simulink model "FOC_PIL_StateMch_top"  (R2020b)
settings: Solver=FixedStepAuto  StartTime=0.0  StopTime=4  FixedStep=Ts_simscape  RelTol=1e-3
values from neighbouring files (symbols this model uses):
  Tctr = 0.0000625    (= 6.25e-05)    [FOC_Config.m]
undefined symbols (not defined in the file or in its folder): motor, NBits
libraries: fl_lib x51, nesl_utility x15, ee_lib x14, msbAdcArchitectures x4, dspsigops x4, simulink x3
settings Model: Creator=k  LastModifiedBy=k

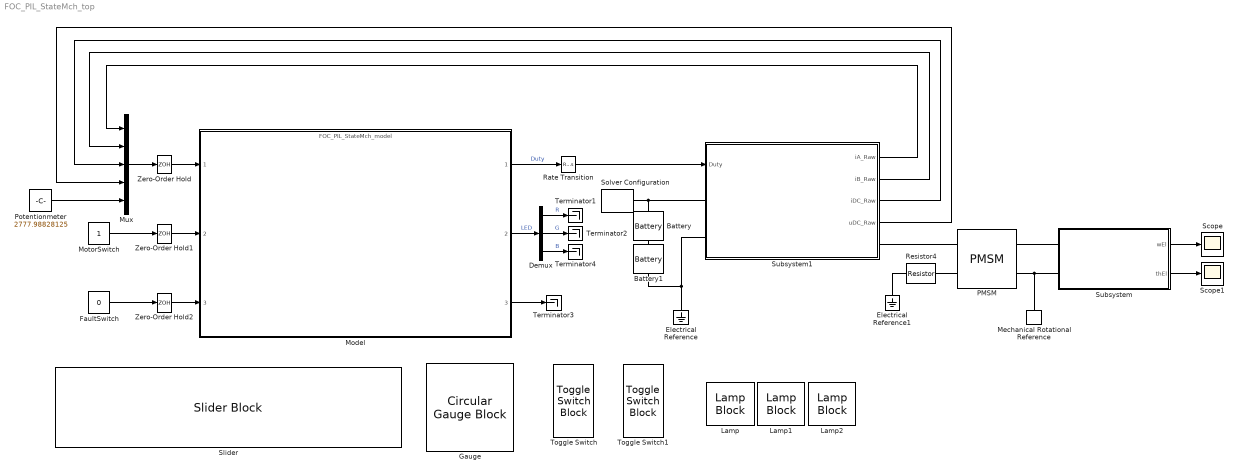
== system FOC_PIL_StateMch_top ==
  Battery : ee_lib/Sources/Battery  Vnom=motor.DC/2 V  prm_dir=1  R1_dis=2 Ohm  R1_ch=2 Ohm  R1=0.2 Ohm  prm_AH=1  AH=50 hr*A  V1=11.5 V  AH1=25 hr*A  prm_R2=1  R2=2000 Ohm  prm_dyn=1  Rp1=0.005 Ohm  tau1=30 s  Rp2=0.005 Ohm  tau2=30 s  Rp3=0.005 Ohm  tau3=30 s  Rp4=0.005 Ohm  tau4=30 s  Rp5=0.005 Ohm  tau5=30 s  prm_fade=1  N_fade=100  AH_fade=45 hr*A  R1_fade=2.02 Ohm  R1_ch_fade=2.02 Ohm  V1_fade=10.35 V  i_specify=off  i_priority=None  i=0 A  i_nominal_specify=off  i_nominal_unit=A  i_nominal_value=1  v_specify=off  v_priority=None  v=0 V  v_nominal_specify=off  v_nominal_unit=V  v_nominal_value=1  charge_specify=off  charge_priority=High  charge=50 hr*A  charge_nominal_specify=off  charge_nominal_unit=hr*A  charge_nominal_value=1  num_cycles_specify=off  num_cycles_priority=High  num_cycles=0  num_cycles_nominal_specify=off  num_cycles_nominal_unit=1  num_cycles_nominal_value=1  thermal_mass=30000 J/K  Tmeas=298.15 K  Vnom_T2=12 V  R1_T2=2.2 Ohm  R1_T2_dis=2.2 Ohm  R1_T2_ch=2.2 Ohm  V1_T2=11.4 V  R2_T2=2200 Ohm  Rp1_T2=0.005 Ohm  tau1_T2=30 s  Rp2_T2=0.005 Ohm  tau2_T2=30 s  Rp3_T2=0.005 Ohm  tau3_T2=30 s  Rp4_T2=0.005 Ohm  tau4_T2=30 s  Rp5_T2=0.005 Ohm  tau5_T2=30 s  Tmeas2=273.15 K  temperature_specify=off  temperature_priority=High  temperature=298.15 K  temperature_nominal_specify=off  temperature_nominal_unit=K  temperature_nominal_value=1
  Battery1 : ee_lib/Sources/Battery  Vnom=motor.DC/2 V  prm_dir=1  R1_dis=2 Ohm  R1_ch=2 Ohm  R1=0.2 Ohm  prm_AH=1  AH=50 hr*A  V1=11.5 V  AH1=25 hr*A  prm_R2=1  R2=2000 Ohm  prm_dyn=1  Rp1=0.005 Ohm  tau1=30 s  Rp2=0.005 Ohm  tau2=30 s  Rp3=0.005 Ohm  tau3=30 s  Rp4=0.005 Ohm  tau4=30 s  Rp5=0.005 Ohm  tau5=30 s  prm_fade=1  N_fade=100  AH_fade=45 hr*A  R1_fade=2.02 Ohm  R1_ch_fade=2.02 Ohm  V1_fade=10.35 V  i_specify=off  i_priority=None  i=0 A  i_nominal_specify=off  i_nominal_unit=A  i_nominal_value=1  v_specify=off  v_priority=None  v=0 V  v_nominal_specify=off  v_nominal_unit=V  v_nominal_value=1  charge_specify=off  charge_priority=High  charge=50 hr*A  charge_nominal_specify=off  charge_nominal_unit=hr*A  charge_nominal_value=1  num_cycles_specify=off  num_cycles_priority=High  num_cycles=0  num_cycles_nominal_specify=off  num_cycles_nominal_unit=1  num_cycles_nominal_value=1  thermal_mass=30000 J/K  Tmeas=298.15 K  Vnom_T2=12 V  R1_T2=2.2 Ohm  R1_T2_dis=2.2 Ohm  R1_T2_ch=2.2 Ohm  V1_T2=11.4 V  R2_T2=2200 Ohm  Rp1_T2=0.005 Ohm  tau1_T2=30 s  Rp2_T2=0.005 Ohm  tau2_T2=30 s  Rp3_T2=0.005 Ohm  tau3_T2=30 s  Rp4_T2=0.005 Ohm  tau4_T2=30 s  Rp5_T2=0.005 Ohm  tau5_T2=30 s  Tmeas2=273.15 K  temperature_specify=off  temperature_priority=High  temperature=298.15 K  temperature_nominal_specify=off  temperature_nominal_unit=K  temperature_nominal_value=1
  Demux : Demux  Outputs=3
  Electrical Reference : fl_lib/Electrical/Electrical Elements/Electrical Reference
  Electrical Reference1 : fl_lib/Electrical/Electrical Elements/Electrical Reference
  FaultSwitch : Constant  Value=0  OutDataTypeStr=boolean
  Gauge : CircularGaugeBlock  ScaleMin=-3.14  ScaleMax=3.14  TickInterval=1.57
  Lamp : LampBlock
  Lamp1 : LampBlock
  Lamp2 : LampBlock
  Mechanical Rotational Reference : fl_lib/Mechanical/Rotational Elements/Mechanical Rotational Reference
  Model : ModelReference  ModelNameDialog=FOC_PIL_StateMch_model.slx  SimulationMode=Processor-in-the-loop (PIL)  ModelReferenceVersion=1.590
  MotorSwitch : Constant  OutDataTypeStr=boolean
  Mux : Mux  Inputs=5
  PMSM : ee_lib/Electromechanical/Permanent Magnet/PMSM  winding_type=ee.enum.statorconnection.wye  machine_param=ee.enum.pmsm.parameterization.constant  nPolePairs=motor.Prs  pmflux_param=ee.enum.pmflux.fluxlinkage  pm_flux_linkage=motor.Flux Wb  torque_constant=0.18 N*m/A  back_emf_constant=0.18 V/(rad/s)  stator_param=ee.enum.statorparam.LdLqL0  Ld=motor.Ld H  Lq=motor.Lq H  idVec=[-200, 0, 200] A  iqVec=[-200, 0, 200] A  LdMatrix=0.0002 * ones(3, 3) H  LqMatrix=0.0002 * ones(3, 3) H  PmMatrix=0.1 * ones(3, 3) Wb  ktMatrix=0.18 * ones(3, 3) N*m/A  keMatrix=0.18 * ones(3, 3) V/(rad/s)  L0=motor.L0 H  Ls=0.0002 H  Lm=-0.00002 H  Ms=0.00002 H  Rs=motor.Rs Ohm  zero_sequence=ee.enum.park.zerosequence.exclude  J=motor.J kg*m^2  lam=motor.B N*m/(rad/s)  axes_param=ee.enum.rotorangle.daxis  i_d_specify=off  i_d_priority=None  i_d=0 A  i_d_nominal_specify=off  i_d_nominal_unit=A  i_d_nominal_value=1  i_q_specify=off  i_q_priority=None  i_q=0 A  i_q_nominal_specify=off  i_q_nominal_unit=A  i_q_nominal_value=1  torque_specify=off  torque_priority=None  torque=0 N*m  torque_nominal_specify=off  torque_nominal_unit=N*m  torque_nominal_value=1  angular_velocity_specify=off  angular_velocity_priority=High  angular_velocity=0 rpm  angular_velocity_nominal_specify=off  angular_velocity_nominal_unit=rpm  angular_velocity_nominal_value=1  angular_position_specify=off  angular_position_priority=High  angular_position=0 deg  angular_position_nominal_specify=off  angular_position_nominal_unit=deg  angular_position_nominal_value=1  loss_param=ee.enum.ironloss.none  losses_oc=[0, 0, 0] W  losses_sc=[0, 0, 0] W  f_losses=60 Hz  Isc_losses=95 A  Tmeas=298.15 K  alpha=3.93e-3 1/K  alpha_flux=-0.001 1/K  stator_thermal_mass=100 J/K  rotor_thermal_mass=200 J/K  Rm_percent_rotor=90  Rd_percent_rotor=30  temperatureA_specify=off  temperatureA_priority=High  temperatureA=25 degC  temperatureA_nominal_specify=off  temperatureA_nominal_unit=degC  temperatureA_nominal_value=1  temperatureB_specify=off  temperatureB_priority=High  temperatureB=25 degC  temperatureB_nominal_specify=off  temperatureB_nominal_unit=degC  temperatureB_nominal_value=1  temperatureC_specify=off  temperatureC_priority=High  temperatureC=25 degC  temperatureC_nominal_specify=off  temperatureC_nominal_unit=degC  temperatureC_nominal_value=1  temperatureR_specify=off  temperatureR_priority=High  temperatureR=25 degC  temperatureR_nominal_specify=off  temperatureR_nominal_unit=degC  temperatureR_nominal_value=1
      settings: InternalSimscapePortConfiguration="{\"Bottom\":[],\"Left\":[{\"id\":\"N\",\"label\":\"~\",\"type\":\"foundation.electrical.three_phase\"},{\"id\":\"n\",\"label\":\"n\",\"type\":\"foundation.electrical.electrical\"}],\"Right\":[{\"id\":\"R\",\"label\":\"R\",\"type\":\"foundation.mechanical.rotational.rotational\"},{\"id\":\"C\",\"label\":\"C\",\"type\":\"foundation.mechanical.rotational.rotational\"}],\"Top\":[]}"
  Potentionmeter : Constant  Value=2777.98828125  OutDataTypeStr=uint16
  Rate Transition : RateTransition
  Resistor4 : fl_lib/Electrical/Electrical Elements/Resistor  R=1e6 Ohm  i_specify=off  i_priority=None  i=0 A  i_nominal_specify=off  i_nominal_unit=A  i_nominal_value=1  v_specify=off  v_priority=None  v=0 V  v_nominal_specify=off  v_nominal_unit=V  v_nominal_value=1
  Scope : Scope
  Scope1 : Scope
  Slider : SliderBlock  ScaleMax=4095
  Solver Configuration : nesl_utility/Solver Configuration  PhysicalDomain=network_engine_domain  SubClassName=solver  LeftPortType=input  RightPortType=generic  Tones=[]  Harmonics=[]  SimulateNoise=off  Profile=off  UseLocalSampling=off  EnableSwitchedLinearOptims=on  FrequencyDomain=off  UseCCode=off  RelTol=0.001  AbsTol=1e-06  MinStep=1e-09  ToWorkspace=off  RevertToSquareIcSolve=off  NumHomotopyIterations=100  PhasorMode=off  PhasorModeNumHarmonics=1  DoDC=off  ResidualTolerance=1e-09  UseLocalSolver=off  LocalSolverChoice=NE_BACKWARD_EULER_ADVANCER  LocalSolverSampleTime=0.001  DoFixedCost=off  MaxNonlinIter=3  MaxModeIter=2  ComputeImpulses=off  ImpulseIterations=2  LinearAlgebra=auto  EquationFormulation=NE_TIME_EF  DelaysMemoryBudget=1024  AutomaticFiltering=on  FilteringTimeConstant=0.001  PartitionStorageMethod=AS_NEEDED  PartitionMemoryBudget=1024  PartitionMethod=ROBUST
  Subsystem : Subsystem
  Subsystem1 : Subsystem
  Terminator{1..4} (4 alike) : Terminator
  Toggle Switch : ToggleSwitchBlock
      settings: Values={{'Off', 'On'}, [0 1]}
  Toggle Switch1 : ToggleSwitchBlock
      settings: Values={{'Off', 'On'}, [0 1]}
  Zero-Order Hold : ZeroOrderHold  SampleTime=Tctr
  Zero-Order Hold1 : ZeroOrderHold  SampleTime=Tctr
  Zero-Order Hold2 : ZeroOrderHold  SampleTime=Tctr
  wires:
  Model/2 -> Demux/1  "LED"
  Model/3 -> Terminator3/1
  Model/1 -> Rate Transition/1  "Duty"
  Subsystem1/3(" iDC_Raw") -> Mux/3
  Mux/1 -> Zero-Order Hold/1
  Subsystem1/1(" iA_Raw") -> Mux/1
  Subsystem1/2(" iB_Raw") -> Mux/2
  Subsystem1/4(" uDC_Raw") -> Mux/4
  Potentionmeter/1 -> Mux/5
  MotorSwitch/1 -> Zero-Order Hold1/1
  FaultSwitch/1 -> Zero-Order Hold2/1
  Zero-Order Hold/1 -> Model/1
  Zero-Order Hold1/1 -> Model/2
  Zero-Order Hold2/1 -> Model/3
  Rate Transition/1 -> Subsystem1/1(Duty)
  Subsystem/1(wEl) -> Scope/1
  Subsystem/2(thEl) -> Scope1/1
  Demux/1 -> Terminator1/1  "R"
  Demux/2 -> Terminator2/1  "G"
  Demux/3 -> Terminator4/1  "B"
  connections:
  Subsystem1/LConn2 -- Electrical Reference/LConn1 -- Battery1/RConn1
  Subsystem1/LConn1 -- Solver Configuration/RConn1 -- Battery/LConn1
  Resistor4/RConn1 -- Electrical Reference1/LConn1
  Resistor4/LConn1 -- PMSM/LConn2
  Battery1/LConn1 -- Battery/RConn1
  PMSM/RConn2 -- Mechanical Rotational Reference/LConn1 -- Subsystem/LConn2
  Subsystem1/RConn1 -- PMSM/LConn1
  Subsystem/LConn1 -- PMSM/RConn1

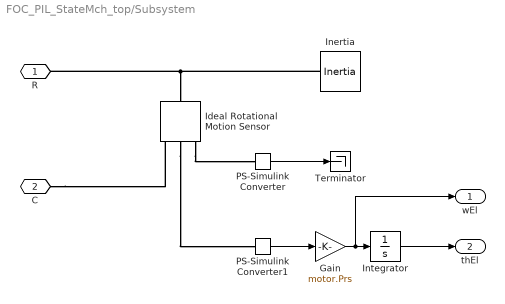
== system FOC_PIL_StateMch_top/Subsystem ==
  Gain : Gain  Gain=motor.Prs
  Ideal Rotational Motion Sensor : fl_lib/Mechanical/Mechanical Sensors/Ideal Rotational Motion Sensor  wrap_angle=simscape.enum.onoff.on  offset=0 rad
  Inertia : fl_lib/Mechanical/Rotational Elements/Inertia  inertia=0.000001 kg*m^2  num_ports=foundation.enum.numPorts2.one  w_specify=off  w_priority=High  w=0 rad/s  w_nominal_specify=off  w_nominal_unit=rad/s  w_nominal_value=1  t_specify=off  t_priority=None  t=0 N*m  t_nominal_specify=off  t_nominal_unit=N*m  t_nominal_value=1
  Integrator : Integrator  WrapState=on
  PS-Simulink Converter : nesl_utility/PS-Simulink Converter  PhysicalDomain=network_engine_domain  SubClassName=ps_output  LeftPortType=input  RightPortType=output  PseudoPeriodic=off  Frequencies=[]  Unit=inherit  AffineConversion=off
  PS-Simulink Converter1 : nesl_utility/PS-Simulink Converter  PhysicalDomain=network_engine_domain  SubClassName=ps_output  LeftPortType=input  RightPortType=output  PseudoPeriodic=off  Frequencies=[]  Unit=inherit  AffineConversion=off
  Terminator : Terminator
  R : PMIOPort  Side=Left
  C : PMIOPort  Port=2  Side=Left
  wEl : Outport
  thEl : Outport  Port=2
  wires:
  PS-Simulink Converter1/1 -> Gain/1
  Integrator/1 -> thEl/1
  PS-Simulink Converter/1 -> Terminator/1
  Gain/1 -> wEl/1, Integrator/1
  connections:
  C/RConn1 -- Ideal Rotational Motion Sensor/RConn1
  Inertia/LConn1 -- R/RConn1 -- Ideal Rotational Motion Sensor/LConn1
  Ideal Rotational Motion Sensor/RConn2 -- PS-Simulink Converter1/LConn1
  Ideal Rotational Motion Sensor/RConn3 -- PS-Simulink Converter/LConn1

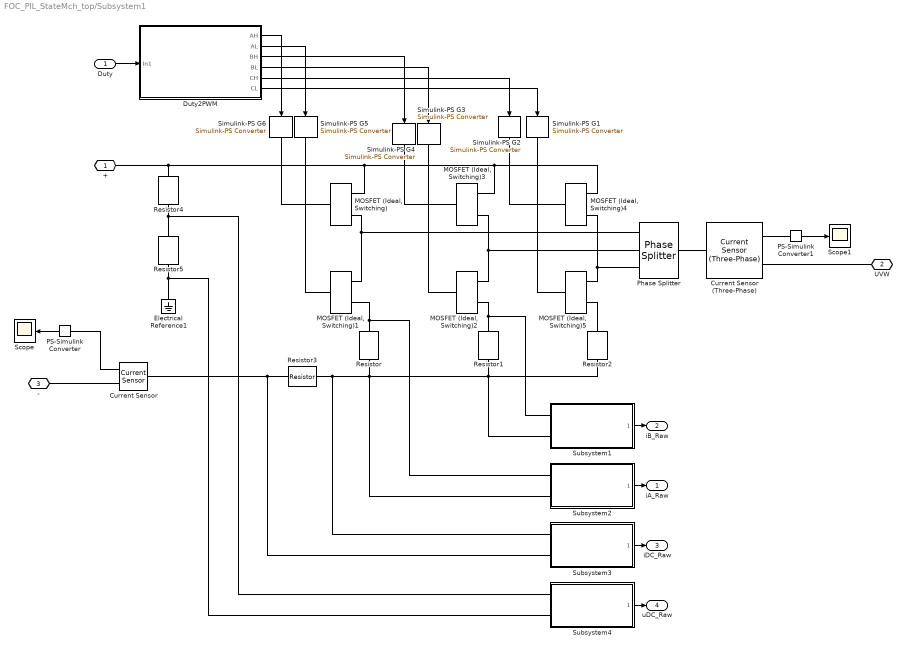
== system FOC_PIL_StateMch_top/Subsystem1 ==
  Duty : Inport
  Current Sensor : fl_lib/Electrical/Electrical Sensors/Current Sensor
  Current Sensor (Three-Phase) : ee_lib/Sensors & Transducers/Current Sensor (Three-Phase)
  Duty2PWM : Subsystem
  Electrical Reference1 : fl_lib/Electrical/Electrical Elements/Electrical Reference
  MOSFET (Ideal, Switching){,1..5} (6 alike) : ee_lib/Semiconductors & Converters/MOSFET (Ideal, Switching)  Rds=0.035 Ohm  Goff=1e-6 1/Ohm  Vth=0.5 V  diode_param=1  diode_Vf=0.8 V  diode_Ron=0.001 Ohm  diode_Goff=1e-5 1/Ohm  diode_C=50e-9 F  diode_iRM=-235 A  diode_iF=300 A  diode_idot=-50 A/us  diode_trr_param=1  diode_trr_factor=3  diode_trr=15 us  diode_Qrr=1500 s*uA  thermal_loss_option=ee.enum.converters.thermalLossOption.constantvalues  Von_data=[0, 1.1, 1.3, 1.45, 1.75, 2.25, 2.7; 0, 1, 1.15, 1.35, 1.7, 2.35, 3] V  Eon_data=[0, .29, 1.43, 2.86, 5.71, 13.14, 22.86; 0, .57, 2.63, 5.14, 10.29, 20.57, 30.29] * 1e-3 J  Eoff_data=[0, .21, 1.07, 2.14, 4.29, 9.86, 17.14; 0, .43, 1.97, 3.86, 7.71, 15.43, 22.71] * 1e-3 J  Tj=[298.15, 398.15] K  Iout_data=[0, 10, 50, 100, 200, 400, 600] A  Eon_scalar=22.86e-3 J  Eoff_scalar=17.14e-3 J  Voff=300 V  Iout_scalar=600 A  diodeModelType=ee.enum.converters.diodeModelType.pwl  diode_IfMat=[.07, .12, .19, 1.75, 4.24, 7.32, 11.2; .16, .3, .72, 2.14, 4.02, 6.35, 9.12] A  diode_TjVec=[25, 125] degC  diode_VfVec=[.5, .7, .9, 1.3, 1.7, 2.1, 2.5] V  thermal_network_parameterization=ee.enum.thermalNetworkTopology.external  Rth=[.03, .2] K/W  Rth_Foster=[.03, .2] K/W  thermal_mass_parameterization=ee.enum.thermalNetwork.timeconstant  thermal_mass=[3, 25] J/K  thermal_mass_Foster=[33, 50] J/K  thermal_time_constant=[.1, 5] s  thermal_time_constant_Foster=[1, 10] s  thermal_mass_initial_temperatures=[25, 25] degC  junction_thermal_mass=0.1 J/K  Tau=1e-4 s  vT_specify=off  vT_priority=None  vT=0 V  vT_nominal_specify=off  vT_nominal_unit=V  vT_nominal_value=1  Qj_specify=off  Qj_priority=None  Qj=0 W  Qj_nominal_specify=off  Qj_nominal_unit=W  Qj_nominal_value=1  junction_temperature_specify=off  junction_temperature_priority=None  junction_temperature=25 degC  junction_temperature_nominal_specify=off  junction_temperature_nominal_unit=degC  junction_temperature_nominal_value=1
  PS-Simulink Converter : nesl_utility/PS-Simulink Converter  PhysicalDomain=network_engine_domain  SubClassName=ps_output  LeftPortType=input  RightPortType=output  PseudoPeriodic=off  Frequencies=[]  Unit=inherit  AffineConversion=off
  PS-Simulink Converter1 : nesl_utility/PS-Simulink Converter  PhysicalDomain=network_engine_domain  SubClassName=ps_output  LeftPortType=input  RightPortType=output  PseudoPeriodic=off  Frequencies=[]  Unit=inherit  AffineConversion=off
  Phase Splitter : ee_lib/Connectors & References/Phase Splitter
      settings: SourceProductBaseCode=PS
  Resistor{,1..3} (4 alike) : fl_lib/Electrical/Electrical Elements/Resistor  R=0.01 Ohm  i_specify=off  i_priority=None  i=0 A  i_nominal_specify=off  i_nominal_unit=A  i_nominal_value=1  v_specify=off  v_priority=None  v=0 V  v_nominal_specify=off  v_nominal_unit=V  v_nominal_value=1
  Resistor4 : fl_lib/Electrical/Electrical Elements/Resistor  R=24000 Ohm  i_specify=off  i_priority=None  i=0 A  i_nominal_specify=off  i_nominal_unit=A  i_nominal_value=1  v_specify=off  v_priority=None  v=0 V  v_nominal_specify=off  v_nominal_unit=V  v_nominal_value=1
  Resistor5 : fl_lib/Electrical/Electrical Elements/Resistor  R=3000 Ohm  i_specify=off  i_priority=None  i=0 A  i_nominal_specify=off  i_nominal_unit=A  i_nominal_value=1  v_specify=off  v_priority=None  v=0 V  v_nominal_specify=off  v_nominal_unit=V  v_nominal_value=1
  Scope : Scope
  Scope1 : Scope
  Simulink-PS G{1..6} (6 alike) : nesl_utility/Simulink-PS Converter  PhysicalDomain=network_engine_domain  SubClassName=ps_input  LeftPortType=input  RightPortType=output  PseudoPeriodic=off  Frequencies=[]  NoiseDistribution=none  NoiseParameters=[]  Unit=1  AffineConversion=off  FilteringAndDerivatives=zero  SimscapeFilterOrder=1  InputFilterTimeConstant=1e-6  UdotUserProvided=0
      settings: SourceProductName=Utilities
  Subsystem1 : Subsystem
  Subsystem2 : Subsystem
  Subsystem3 : Subsystem
  Subsystem4 : Subsystem
  + : PMIOPort  Side=Left
  UVW : PMIOPort  Port=2  Side=Right
  - : PMIOPort  Port=3  Side=Left
  " iA_Raw" : Outport
  " iB_Raw" : Outport  Port=2
  " iDC_Raw" : Outport  Port=3
  " uDC_Raw" : Outport  Port=4
  wires:
  Subsystem3/1(" ") -> " iDC_Raw"/1
  Subsystem2/1(" ") -> " iA_Raw"/1
  Subsystem1/1(" ") -> " iB_Raw"/1
  Duty/1 -> Duty2PWM/1(In1)
  Duty2PWM/1(AH) -> Simulink-PS G6/1
  Duty2PWM/2(AL) -> Simulink-PS G5/1
  Duty2PWM/3(BH) -> Simulink-PS G4/1
  Duty2PWM/4(BL) -> Simulink-PS G3/1
  Duty2PWM/5(CH) -> Simulink-PS G2/1
  Duty2PWM/6(CL) -> Simulink-PS G1/1
  PS-Simulink Converter/1 -> Scope/1
  PS-Simulink Converter1/1 -> Scope1/1
  Subsystem4/1(" ") -> " uDC_Raw"/1
  connections:
  Subsystem3/LConn2 -- Resistor3/RConn1 -- Current Sensor/LConn1
  Simulink-PS G3/RConn1 -- "MOSFET (Ideal, Switching)2"/LConn1
  "MOSFET (Ideal, Switching)4"/RConn2 -- "MOSFET (Ideal, Switching)5"/RConn1 -- Phase Splitter/RConn3
  Phase Splitter/RConn1 -- "MOSFET (Ideal, Switching)"/RConn2 -- "MOSFET (Ideal, Switching)1"/RConn1
  Simulink-PS G4/RConn1 -- "MOSFET (Ideal, Switching)3"/LConn1
  Subsystem2/LConn2 -- Subsystem1/LConn2 -- Resistor1/RConn1 -- Resistor2/RConn1 -- Resistor/RConn1 -- Resistor3/LConn1 -- Subsystem3/LConn1
  "MOSFET (Ideal, Switching)2"/RConn2 -- Subsystem1/LConn1 -- Resistor1/LConn1
  +/RConn1 -- "MOSFET (Ideal, Switching)"/RConn1 -- "MOSFET (Ideal, Switching)3"/RConn1 -- "MOSFET (Ideal, Switching)4"/RConn1 -- Resistor4/LConn1
  Phase Splitter/RConn2 -- "MOSFET (Ideal, Switching)3"/RConn2 -- "MOSFET (Ideal, Switching)2"/RConn1
  Simulink-PS G6/RConn1 -- "MOSFET (Ideal, Switching)"/LConn1
  "MOSFET (Ideal, Switching)1"/RConn2 -- Resistor/LConn1 -- Subsystem2/LConn1
  Simulink-PS G2/RConn1 -- "MOSFET (Ideal, Switching)4"/LConn1
  Simulink-PS G5/RConn1 -- "MOSFET (Ideal, Switching)1"/LConn1
  "MOSFET (Ideal, Switching)5"/RConn2 -- Resistor2/LConn1
  Simulink-PS G1/RConn1 -- "MOSFET (Ideal, Switching)5"/LConn1
  Current Sensor (Three-Phase)/LConn1 -- Phase Splitter/LConn1
  Current Sensor/RConn2 -- -/RConn1
  Current Sensor/RConn1 -- PS-Simulink Converter/LConn1
  Current Sensor (Three-Phase)/RConn2 -- UVW/RConn1
  Current Sensor (Three-Phase)/RConn1 -- PS-Simulink Converter1/LConn1
  Resistor5/LConn1 -- Subsystem4/LConn1 -- Resistor4/RConn1
  Electrical Reference1/LConn1 -- Resistor5/RConn1 -- Subsystem4/LConn2

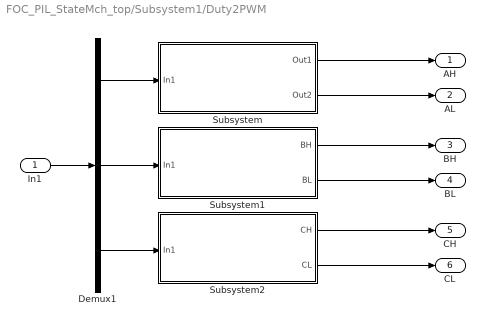
== system FOC_PIL_StateMch_top/Subsystem1/Duty2PWM ==
  In1 : Inport
  Demux1 : Demux  Outputs=3
  Subsystem : Subsystem
  Subsystem1 : Subsystem
  Subsystem2 : Subsystem
  AH : Outport
  AL : Outport  Port=2
  BH : Outport  Port=3
  BL : Outport  Port=4
  CH : Outport  Port=5
  CL : Outport  Port=6
  wires:
  Demux1/1 -> Subsystem/1(In1)
  Demux1/3 -> Subsystem2/1(In1)
  Demux1/2 -> Subsystem1/1(In1)
  In1/1 -> Demux1/1
  Subsystem/1(Out1) -> AH/1
  Subsystem/2(Out2) -> AL/1
  Subsystem1/1(BH) -> BH/1
  Subsystem1/2(BL) -> BL/1
  Subsystem2/1(CH) -> CH/1
  Subsystem2/2(CL) -> CL/1

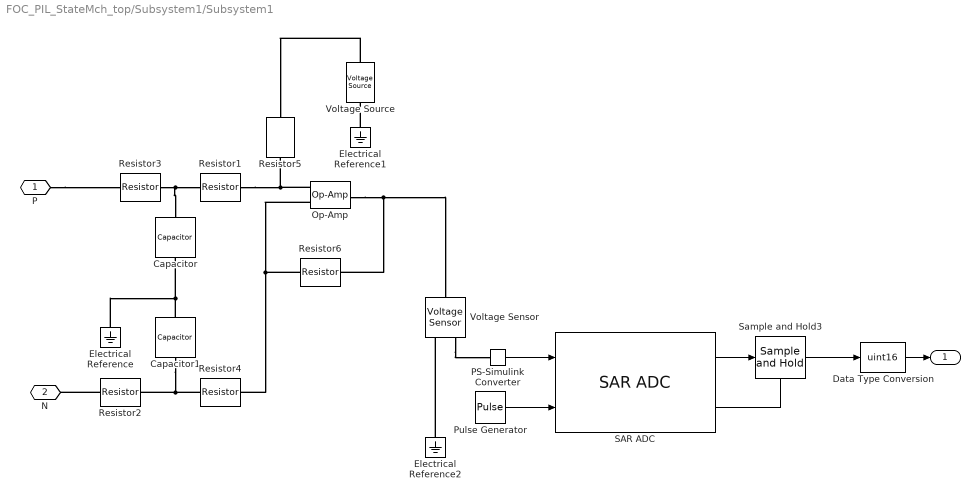
== system FOC_PIL_StateMch_top/Subsystem1/Subsystem1 ==
  Capacitor : fl_lib/Electrical/Electrical Elements/Capacitor  c=47 pF  r=1e-6 Ohm  g=0 1/Ohm  i_specify=off  i_priority=None  i=0 A  i_nominal_specify=off  i_nominal_unit=A  i_nominal_value=1  v_specify=off  v_priority=None  v=0 V  v_nominal_specify=off  v_nominal_unit=V  v_nominal_value=1  vc_specify=off  vc_priority=High  vc=0 V  vc_nominal_specify=off  vc_nominal_unit=V  vc_nominal_value=1
  Capacitor1 : fl_lib/Electrical/Electrical Elements/Capacitor  c=47 pF  r=1e-6 Ohm  g=0 1/Ohm  i_specify=off  i_priority=None  i=0 A  i_nominal_specify=off  i_nominal_unit=A  i_nominal_value=1  v_specify=off  v_priority=None  v=0 V  v_nominal_specify=off  v_nominal_unit=V  v_nominal_value=1  vc_specify=off  vc_priority=High  vc=0 V  vc_nominal_specify=off  vc_nominal_unit=V  vc_nominal_value=1
  Data Type Conversion : DataTypeConversion  OutDataTypeStr=uint16
  Electrical Reference : fl_lib/Electrical/Electrical Elements/Electrical Reference
  Electrical Reference1 : fl_lib/Electrical/Electrical Elements/Electrical Reference
  Electrical Reference2 : fl_lib/Electrical/Electrical Elements/Electrical Reference
  Op-Amp : fl_lib/Electrical/Electrical Elements/Op-Amp  outI_specify=off  outI_priority=None  outI=0 A  outI_nominal_specify=off  outI_nominal_unit=A  outI_nominal_value=1
  PS-Simulink Converter : nesl_utility/PS-Simulink Converter  PhysicalDomain=network_engine_domain  SubClassName=ps_output  LeftPortType=input  RightPortType=output  PseudoPeriodic=off  Frequencies=[]  Unit=inherit  AffineConversion=off
  Pulse Generator : DiscretePulseGenerator  PulseType=Time based  Period=Tctr  PulseWidth=50  PhaseDelay=Tctr
  Resistor{1..4} (4 alike) : fl_lib/Electrical/Electrical Elements/Resistor  R=1500 Ohm  i_specify=off  i_priority=None  i=0 A  i_nominal_specify=off  i_nominal_unit=A  i_nominal_value=1  v_specify=off  v_priority=None  v=0 V  v_nominal_specify=off  v_nominal_unit=V  v_nominal_value=1
  Resistor5 : fl_lib/Electrical/Electrical Elements/Resistor  R=24000 Ohm  i_specify=off  i_priority=None  i=0 A  i_nominal_specify=off  i_nominal_unit=A  i_nominal_value=1  v_specify=off  v_priority=None  v=0 V  v_nominal_specify=off  v_nominal_unit=V  v_nominal_value=1
  Resistor6 : fl_lib/Electrical/Electrical Elements/Resistor  R=24000 Ohm  i_specify=off  i_priority=None  i=0 A  i_nominal_specify=off  i_nominal_unit=A  i_nominal_value=1  v_specify=off  v_priority=None  v=0 V  v_nominal_specify=off  v_nominal_unit=V  v_nominal_value=1
  SAR ADC : msbAdcArchitectures/SAR ADC  DACVoltages=[-5:5]  DACINLVoltages=tanh([-5:5])  NBits=12  InputRange=[0 5]  ExtStartClk=on  StartFreq=10e3  StartClkJitter=0  SARFreq=2e6  MatchScale=off  OutputPolarity=Auto  OutDataType=fixdt(0,NBits)  EnableImp=off  OffsetError=1  OffsetErrorUnit=LSB  GainError=2  GainErrorUnit=LSB
      settings: SourceProductBaseCode=AM
  Sample and Hold3 : dspsigops/Sample and Hold  trig=Rising edge  initCond=0  latchinput=off
  Voltage Sensor : fl_lib/Electrical/Electrical Sensors/Voltage Sensor
  Voltage Source : ee_lib/Sources/Voltage Source  dc_voltage=2.5 V  ac_voltage=0 V  ac_shift=0 rad  ac_frequency=60 Hz  noise_mode=0  PSD=0 V^2/Hz  repeatability=1  auto_seed=3922919431  user_seed=0  sample_time=1e-3 s  i_specify=off  i_priority=None  i=0 A  i_nominal_specify=off  i_nominal_unit=A  i_nominal_value=1  v_specify=off  v_priority=None  v=0 V  v_nominal_specify=off  v_nominal_unit=V  v_nominal_value=1
  P : PMIOPort  Side=Left
  N : PMIOPort  Port=2  Side=Left
  " " : Outport
  wires:
  Pulse Generator/1 -> SAR ADC/2
  Data Type Conversion/1 -> " "/1
  PS-Simulink Converter/1 -> SAR ADC/1
  SAR ADC/1 -> Sample and Hold3/1
  Sample and Hold3/1 -> Data Type Conversion/1
  SAR ADC/2 -> Sample and Hold3/Trigger
  connections:
  Voltage Sensor/RConn1 -- PS-Simulink Converter/LConn1
  Resistor2/LConn1 -- N/RConn1
  P/RConn1 -- Resistor3/LConn1
  Resistor3/RConn1 -- Capacitor/LConn1 -- Resistor1/LConn1
  Resistor1/RConn1 -- Resistor5/RConn1 -- Op-Amp/LConn1
  Capacitor/RConn1 -- Capacitor1/LConn1 -- Electrical Reference/LConn1
  Resistor2/RConn1 -- Resistor4/LConn1 -- Capacitor1/RConn1
  Resistor4/RConn1 -- Resistor6/LConn1 -- Op-Amp/LConn2
  Voltage Source/LConn1 -- Resistor5/LConn1
  Electrical Reference1/LConn1 -- Voltage Source/RConn1
  Resistor6/RConn1 -- Voltage Sensor/LConn1 -- Op-Amp/RConn1
  Electrical Reference2/LConn1 -- Voltage Sensor/RConn2

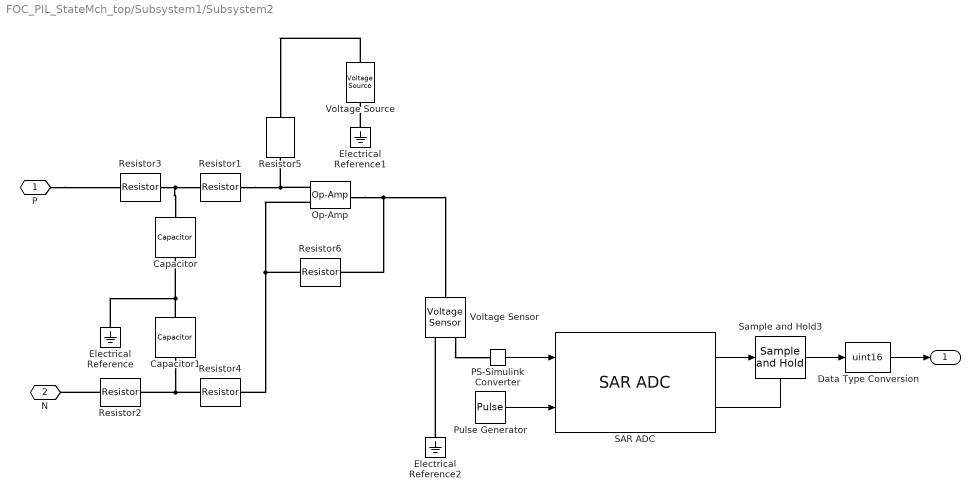
== system FOC_PIL_StateMch_top/Subsystem1/Subsystem2 ==
  Capacitor : fl_lib/Electrical/Electrical Elements/Capacitor  c=47 pF  r=1e-6 Ohm  g=0 1/Ohm  i_specify=off  i_priority=None  i=0 A  i_nominal_specify=off  i_nominal_unit=A  i_nominal_value=1  v_specify=off  v_priority=None  v=0 V  v_nominal_specify=off  v_nominal_unit=V  v_nominal_value=1  vc_specify=off  vc_priority=High  vc=0 V  vc_nominal_specify=off  vc_nominal_unit=V  vc_nominal_value=1
  Capacitor1 : fl_lib/Electrical/Electrical Elements/Capacitor  c=47 pF  r=1e-6 Ohm  g=0 1/Ohm  i_specify=off  i_priority=None  i=0 A  i_nominal_specify=off  i_nominal_unit=A  i_nominal_value=1  v_specify=off  v_priority=None  v=0 V  v_nominal_specify=off  v_nominal_unit=V  v_nominal_value=1  vc_specify=off  vc_priority=High  vc=0 V  vc_nominal_specify=off  vc_nominal_unit=V  vc_nominal_value=1
  Data Type Conversion : DataTypeConversion  OutDataTypeStr=uint16
  Electrical Reference : fl_lib/Electrical/Electrical Elements/Electrical Reference
  Electrical Reference1 : fl_lib/Electrical/Electrical Elements/Electrical Reference
  Electrical Reference2 : fl_lib/Electrical/Electrical Elements/Electrical Reference
  Op-Amp : fl_lib/Electrical/Electrical Elements/Op-Amp  outI_specify=off  outI_priority=None  outI=0 A  outI_nominal_specify=off  outI_nominal_unit=A  outI_nominal_value=1
  PS-Simulink Converter : nesl_utility/PS-Simulink Converter  PhysicalDomain=network_engine_domain  SubClassName=ps_output  LeftPortType=input  RightPortType=output  PseudoPeriodic=off  Frequencies=[]  Unit=inherit  AffineConversion=off
  Pulse Generator : DiscretePulseGenerator  PulseType=Time based  Period=Tctr  PulseWidth=50  PhaseDelay=Tctr
  Resistor{1..4} (4 alike) : fl_lib/Electrical/Electrical Elements/Resistor  R=1500 Ohm  i_specify=off  i_priority=None  i=0 A  i_nominal_specify=off  i_nominal_unit=A  i_nominal_value=1  v_specify=off  v_priority=None  v=0 V  v_nominal_specify=off  v_nominal_unit=V  v_nominal_value=1
  Resistor5 : fl_lib/Electrical/Electrical Elements/Resistor  R=24000 Ohm  i_specify=off  i_priority=None  i=0 A  i_nominal_specify=off  i_nominal_unit=A  i_nominal_value=1  v_specify=off  v_priority=None  v=0 V  v_nominal_specify=off  v_nominal_unit=V  v_nominal_value=1
  Resistor6 : fl_lib/Electrical/Electrical Elements/Resistor  R=24000 Ohm  i_specify=off  i_priority=None  i=0 A  i_nominal_specify=off  i_nominal_unit=A  i_nominal_value=1  v_specify=off  v_priority=None  v=0 V  v_nominal_specify=off  v_nominal_unit=V  v_nominal_value=1
  SAR ADC : msbAdcArchitectures/SAR ADC  DACVoltages=[-5:5]  DACINLVoltages=tanh([-5:5])  NBits=12  InputRange=[0 5]  ExtStartClk=on  StartFreq=10e3  StartClkJitter=0  SARFreq=2e6  MatchScale=off  OutputPolarity=Auto  OutDataType=fixdt(0,NBits)  EnableImp=off  OffsetError=1  OffsetErrorUnit=LSB  GainError=2  GainErrorUnit=LSB
      settings: SourceProductBaseCode=AM
  Sample and Hold3 : dspsigops/Sample and Hold  trig=Rising edge  initCond=0  latchinput=off
  Voltage Sensor : fl_lib/Electrical/Electrical Sensors/Voltage Sensor
  Voltage Source : ee_lib/Sources/Voltage Source  dc_voltage=2.5 V  ac_voltage=0 V  ac_shift=0 rad  ac_frequency=60 Hz  noise_mode=0  PSD=0 V^2/Hz  repeatability=1  auto_seed=2715962282  user_seed=0  sample_time=1e-3 s  i_specify=off  i_priority=None  i=0 A  i_nominal_specify=off  i_nominal_unit=A  i_nominal_value=1  v_specify=off  v_priority=None  v=0 V  v_nominal_specify=off  v_nominal_unit=V  v_nominal_value=1
  P : PMIOPort  Side=Left
  N : PMIOPort  Port=2  Side=Left
  " " : Outport
  wires:
  Data Type Conversion/1 -> " "/1
  PS-Simulink Converter/1 -> SAR ADC/1
  SAR ADC/2 -> Sample and Hold3/Trigger
  SAR ADC/1 -> Sample and Hold3/1
  Pulse Generator/1 -> SAR ADC/2
  Sample and Hold3/1 -> Data Type Conversion/1
  connections:
  Electrical Reference2/LConn1 -- Voltage Sensor/RConn2
  Op-Amp/RConn1 -- Voltage Sensor/LConn1 -- Resistor6/RConn1
  Electrical Reference1/LConn1 -- Voltage Source/RConn1
  Voltage Source/LConn1 -- Resistor5/LConn1
  Op-Amp/LConn2 -- Resistor6/LConn1 -- Resistor4/RConn1
  Capacitor1/RConn1 -- Resistor4/LConn1 -- Resistor2/RConn1
  Electrical Reference/LConn1 -- Capacitor1/LConn1 -- Capacitor/RConn1
  Op-Amp/LConn1 -- Resistor5/RConn1 -- Resistor1/RConn1
  Resistor3/RConn1 -- Resistor1/LConn1 -- Capacitor/LConn1
  P/RConn1 -- Resistor3/LConn1
  Resistor2/LConn1 -- N/RConn1
  Voltage Sensor/RConn1 -- PS-Simulink Converter/LConn1

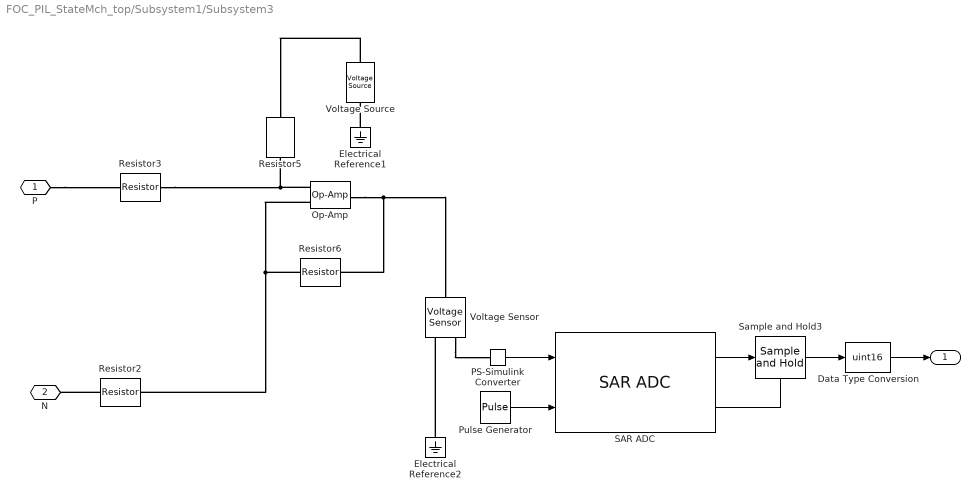
== system FOC_PIL_StateMch_top/Subsystem1/Subsystem3 ==
  Data Type Conversion : DataTypeConversion  OutDataTypeStr=uint16
  Electrical Reference1 : fl_lib/Electrical/Electrical Elements/Electrical Reference
  Electrical Reference2 : fl_lib/Electrical/Electrical Elements/Electrical Reference
  Op-Amp : fl_lib/Electrical/Electrical Elements/Op-Amp  outI_specify=off  outI_priority=None  outI=0 A  outI_nominal_specify=off  outI_nominal_unit=A  outI_nominal_value=1
  PS-Simulink Converter : nesl_utility/PS-Simulink Converter  PhysicalDomain=network_engine_domain  SubClassName=ps_output  LeftPortType=input  RightPortType=output  PseudoPeriodic=off  Frequencies=[]  Unit=inherit  AffineConversion=off
  Pulse Generator : DiscretePulseGenerator  PulseType=Time based  Period=Tctr  PulseWidth=50  PhaseDelay=Tctr/4
  Resistor2 : fl_lib/Electrical/Electrical Elements/Resistor  R=1000 Ohm  i_specify=off  i_priority=None  i=0 A  i_nominal_specify=off  i_nominal_unit=A  i_nominal_value=1  v_specify=off  v_priority=None  v=0 V  v_nominal_specify=off  v_nominal_unit=V  v_nominal_value=1
  Resistor3 : fl_lib/Electrical/Electrical Elements/Resistor  R=1000 Ohm  i_specify=off  i_priority=None  i=0 A  i_nominal_specify=off  i_nominal_unit=A  i_nominal_value=1  v_specify=off  v_priority=None  v=0 V  v_nominal_specify=off  v_nominal_unit=V  v_nominal_value=1
  Resistor5 : fl_lib/Electrical/Electrical Elements/Resistor  R=10000 Ohm  i_specify=off  i_priority=None  i=0 A  i_nominal_specify=off  i_nominal_unit=A  i_nominal_value=1  v_specify=off  v_priority=None  v=0 V  v_nominal_specify=off  v_nominal_unit=V  v_nominal_value=1
  Resistor6 : fl_lib/Electrical/Electrical Elements/Resistor  R=10000 Ohm  i_specify=off  i_priority=None  i=0 A  i_nominal_specify=off  i_nominal_unit=A  i_nominal_value=1  v_specify=off  v_priority=None  v=0 V  v_nominal_specify=off  v_nominal_unit=V  v_nominal_value=1
  SAR ADC : msbAdcArchitectures/SAR ADC  DACVoltages=[-5:5]  DACINLVoltages=tanh([-5:5])  NBits=12  InputRange=[0 5]  ExtStartClk=on  StartFreq=10e3  StartClkJitter=0  SARFreq=2e6  MatchScale=off  OutputPolarity=Auto  OutDataType=fixdt(0,NBits)  EnableImp=off  OffsetError=1  OffsetErrorUnit=LSB  GainError=2  GainErrorUnit=LSB
      settings: SourceProductBaseCode=AM
  Sample and Hold3 : dspsigops/Sample and Hold  trig=Rising edge  initCond=0  latchinput=off
  Voltage Sensor : fl_lib/Electrical/Electrical Sensors/Voltage Sensor
  Voltage Source : ee_lib/Sources/Voltage Source  dc_voltage=2.5 V  ac_voltage=0 V  ac_shift=0 rad  ac_frequency=60 Hz  noise_mode=0  PSD=0 V^2/Hz  repeatability=1  auto_seed=418932850  user_seed=0  sample_time=1e-3 s  i_specify=off  i_priority=None  i=0 A  i_nominal_specify=off  i_nominal_unit=A  i_nominal_value=1  v_specify=off  v_priority=None  v=0 V  v_nominal_specify=off  v_nominal_unit=V  v_nominal_value=1
  P : PMIOPort  Side=Left
  N : PMIOPort  Port=2  Side=Left
  " " : Outport
  wires:
  Sample and Hold3/1 -> Data Type Conversion/1
  Pulse Generator/1 -> SAR ADC/2
  SAR ADC/1 -> Sample and Hold3/1
  SAR ADC/2 -> Sample and Hold3/Trigger
  PS-Simulink Converter/1 -> SAR ADC/1
  Data Type Conversion/1 -> " "/1
  connections:
  Voltage Sensor/RConn1 -- PS-Simulink Converter/LConn1
  Resistor2/LConn1 -- N/RConn1
  P/RConn1 -- Resistor3/LConn1
  Resistor5/RConn1 -- Op-Amp/LConn1 -- Resistor3/RConn1
  Resistor6/LConn1 -- Op-Amp/LConn2 -- Resistor2/RConn1
  Voltage Source/LConn1 -- Resistor5/LConn1
  Electrical Reference1/LConn1 -- Voltage Source/RConn1
  Resistor6/RConn1 -- Voltage Sensor/LConn1 -- Op-Amp/RConn1
  Electrical Reference2/LConn1 -- Voltage Sensor/RConn2

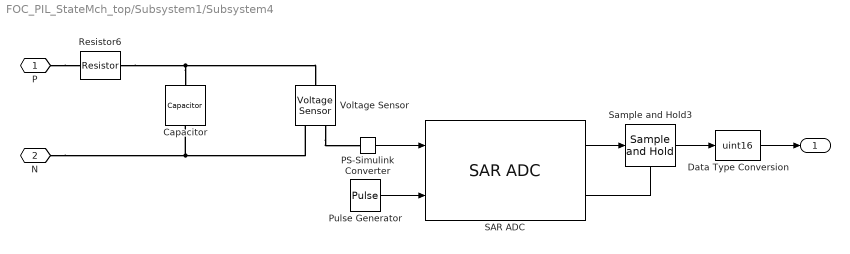
== system FOC_PIL_StateMch_top/Subsystem1/Subsystem4 ==
  Capacitor : fl_lib/Electrical/Electrical Elements/Capacitor  c=82 pF  r=1e-6 Ohm  g=0 1/Ohm  i_specify=off  i_priority=None  i=0 A  i_nominal_specify=off  i_nominal_unit=A  i_nominal_value=1  v_specify=off  v_priority=None  v=0 V  v_nominal_specify=off  v_nominal_unit=V  v_nominal_value=1  vc_specify=off  vc_priority=High  vc=0 V  vc_nominal_specify=off  vc_nominal_unit=V  vc_nominal_value=1
  Data Type Conversion : DataTypeConversion  OutDataTypeStr=uint16
  PS-Simulink Converter : nesl_utility/PS-Simulink Converter  PhysicalDomain=network_engine_domain  SubClassName=ps_output  LeftPortType=input  RightPortType=output  PseudoPeriodic=off  Frequencies=[]  Unit=inherit  AffineConversion=off
  Pulse Generator : DiscretePulseGenerator  PulseType=Time based  Period=Tctr  PulseWidth=50  PhaseDelay=Tctr/2
  Resistor6 : fl_lib/Electrical/Electrical Elements/Resistor  R=120 Ohm  i_specify=off  i_priority=None  i=0 A  i_nominal_specify=off  i_nominal_unit=A  i_nominal_value=1  v_specify=off  v_priority=None  v=0 V  v_nominal_specify=off  v_nominal_unit=V  v_nominal_value=1
  SAR ADC : msbAdcArchitectures/SAR ADC  DACVoltages=[-5:5]  DACINLVoltages=tanh([-5:5])  NBits=12  InputRange=[0 5]  ExtStartClk=on  StartFreq=10e3  StartClkJitter=0  SARFreq=2e6  MatchScale=off  OutputPolarity=Auto  OutDataType=fixdt(0,NBits)  EnableImp=off  OffsetError=1  OffsetErrorUnit=LSB  GainError=2  GainErrorUnit=LSB
      settings: SourceProductBaseCode=AM
  Sample and Hold3 : dspsigops/Sample and Hold  trig=Rising edge  initCond=0  latchinput=off
  Voltage Sensor : fl_lib/Electrical/Electrical Sensors/Voltage Sensor
  P : PMIOPort  Side=Left
  N : PMIOPort  Port=2  Side=Left
  " " : Outport
  wires:
  Data Type Conversion/1 -> " "/1
  PS-Simulink Converter/1 -> SAR ADC/1
  SAR ADC/2 -> Sample and Hold3/Trigger
  SAR ADC/1 -> Sample and Hold3/1
  Pulse Generator/1 -> SAR ADC/2
  Sample and Hold3/1 -> Data Type Conversion/1
  connections:
  Voltage Sensor/RConn1 -- PS-Simulink Converter/LConn1
  Capacitor/LConn1 -- Voltage Sensor/LConn1 -- Resistor6/LConn1
  Voltage Sensor/RConn2 -- Capacitor/RConn1 -- N/RConn1
  P/RConn1 -- Resistor6/RConn1

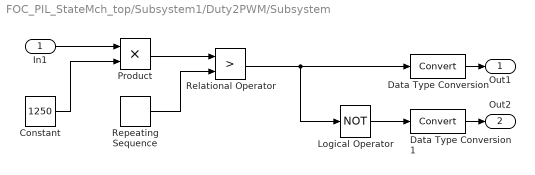
== system FOC_PIL_StateMch_top/Subsystem1/Duty2PWM/Subsystem ==
  In1 : Inport
  Constant : Constant  Value=1250
  Data Type Conversion : DataTypeConversion
  Data Type Conversion1 : DataTypeConversion
  Logical Operator : Logic  Operator=NOT  AllPortsSameDT=off  OutDataTypeStr=boolean
  Product : Product
  Relational Operator : RelationalOperator  Operator=>  OutDataTypeStr=boolean  RndMeth=Simplest
  Repeating Sequence : simulink/Sources/Repeating Sequence  rep_seq_t=[0 1/16000/2 1/16000]  rep_seq_y=[1249 0 1249]
  Out1 : Outport
  Out2 : Outport  Port=2
  wires:
  Repeating Sequence/1 -> Relational Operator/2
  Product/1 -> Relational Operator/1
  Relational Operator/1 -> Logical Operator/1, Data Type Conversion/1
  Constant/1 -> Product/2
  In1/1 -> Product/1
  Logical Operator/1 -> Data Type Conversion1/1
  Data Type Conversion/1 -> Out1/1
  Data Type Conversion1/1 -> Out2/1

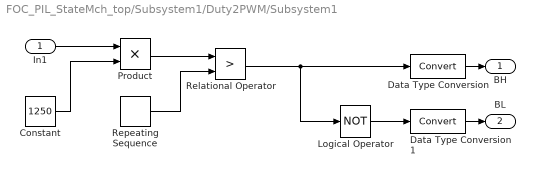
== system FOC_PIL_StateMch_top/Subsystem1/Duty2PWM/Subsystem1 ==
  In1 : Inport
  Constant : Constant  Value=1250
  Data Type Conversion : DataTypeConversion
  Data Type Conversion1 : DataTypeConversion
  Logical Operator : Logic  Operator=NOT  AllPortsSameDT=off  OutDataTypeStr=boolean
  Product : Product
  Relational Operator : RelationalOperator  Operator=>  OutDataTypeStr=boolean  RndMeth=Simplest
  Repeating Sequence : simulink/Sources/Repeating Sequence  rep_seq_t=[0 1/16000/2 1/16000]  rep_seq_y=[1249 0 1249]
  BH : Outport
  BL : Outport  Port=2
  wires:
  Data Type Conversion1/1 -> BL/1
  Data Type Conversion/1 -> BH/1
  Logical Operator/1 -> Data Type Conversion1/1
  In1/1 -> Product/1
  Constant/1 -> Product/2
  Relational Operator/1 -> Data Type Conversion/1, Logical Operator/1
  Product/1 -> Relational Operator/1
  Repeating Sequence/1 -> Relational Operator/2

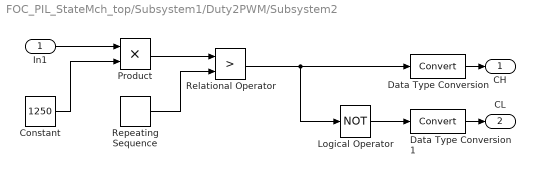
== system FOC_PIL_StateMch_top/Subsystem1/Duty2PWM/Subsystem2 ==
  In1 : Inport
  Constant : Constant  Value=1250
  Data Type Conversion : DataTypeConversion
  Data Type Conversion1 : DataTypeConversion
  Logical Operator : Logic  Operator=NOT  AllPortsSameDT=off  OutDataTypeStr=boolean
  Product : Product
  Relational Operator : RelationalOperator  Operator=>  OutDataTypeStr=boolean  RndMeth=Simplest
  Repeating Sequence : simulink/Sources/Repeating Sequence  rep_seq_t=[0 1/16000/2 1/16000]  rep_seq_y=[1249 0 1249]
  CH : Outport
  CL : Outport  Port=2
  wires:
  Repeating Sequence/1 -> Relational Operator/2
  Product/1 -> Relational Operator/1
  Relational Operator/1 -> Logical Operator/1, Data Type Conversion/1
  Constant/1 -> Product/2
  In1/1 -> Product/1
  Logical Operator/1 -> Data Type Conversion1/1
  Data Type Conversion/1 -> CH/1
  Data Type Conversion1/1 -> CL/1
